simulink subsystem "NoDifferential"  (R2022b)
settings: Solver=VariableStepAuto  StartTime=0.0  StopTime=10.0  RelTol=1e-3
settings Model: Creator=The MathWorks, Inc.  LastModifiedBy=The MathWorks, Inc.

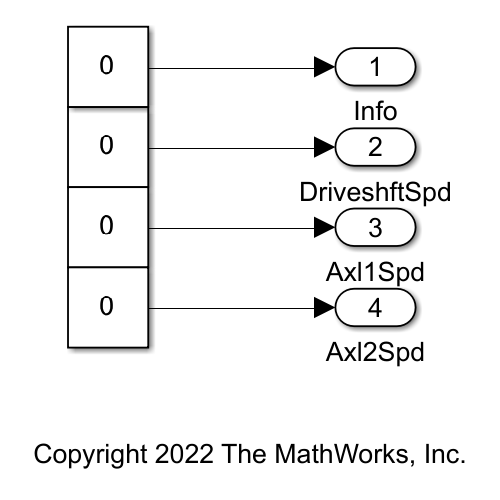
[thumbnail: Simulink's stored preview of the top-level diagram]
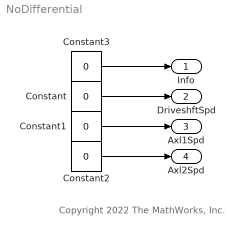
== system NoDifferential ==
  note: Copyright 2022 The MathWorks, Inc.
  Constant{,1..3} (4 alike) : Constant  Value=0  SampleTime=-1
  Info : Outport
  DriveshftSpd : Outport  Port=2
  Axl1Spd : Outport  Port=3
  Axl2Spd : Outport  Port=4
  wires:
  Constant2/1 -> Axl2Spd/1
  Constant1/1 -> Axl1Spd/1
  Constant3/1 -> Info/1
  Constant/1 -> DriveshftSpd/1
